simulink model "FYP_Flywheel_Stage1"  (R2024a)
settings: Solver=ode45  StartTime=0.0  StopTime=10  RelTol=1e-3
values from neighbouring files (symbols this model uses):
  J = 0.5    [FYP_Flywheel_Stage1_build.m]    (also in FYP_Flywheel_Stage2_build.m)
  omega0 = 2*pi*n0/60    (= 314.159265359)    [FYP_Flywheel_Stage1_build.m]    (also in FYP_Flywheel_Stage2_build.m; FYP_Flywheel_Stage3_DCServo_build.m; FYP_Flywheel_Stage4_v2_StableClosedLoop_build.m; FYP_Flywheel_Stage5_COMPLETE_v2.m)
settings Model: Creator=cheng  LastModifiedBy=cheng

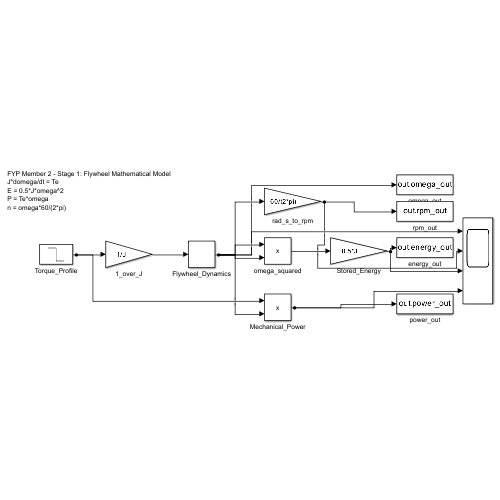
[thumbnail: Simulink's stored preview of the top-level diagram]
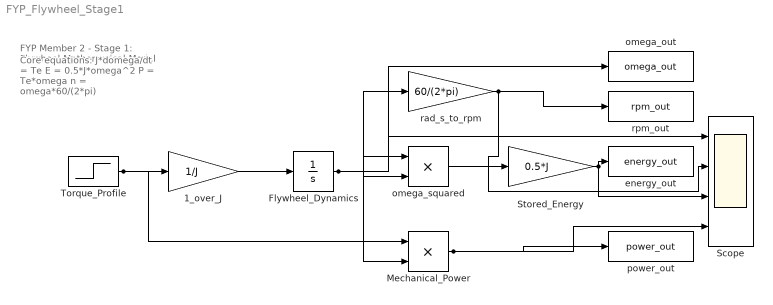
== system FYP_Flywheel_Stage1 ==
  note: FYP Member 2 - Stage 1: Flywheel Mathematical Model
  note: Core equations:
      | J*domega/dt = Te
      | E = 0.5*J*omega^2
      | P = Te*omega
      | n = omega*60/(2*pi)
  1_over_J : Gain  Gain=1/J
  Flywheel_Dynamics : Integrator  InitialCondition=omega0
  Mechanical_Power : Product  Inputs=**
  Scope : Scope  NumInputPorts=4
  Stored_Energy : Gain  Gain=0.5*J
  Torque_Profile : Step  Time=5  Before=5  After=-5  SampleTime=0
  energy_out : ToWorkspace  VariableName=energy_out  SaveFormat=Timeseries  SampleTime=-1
  omega_out : ToWorkspace  VariableName=omega_out  SaveFormat=Timeseries  SampleTime=-1
  omega_squared : Product  Inputs=**
  power_out : ToWorkspace  VariableName=power_out  SaveFormat=Timeseries  SampleTime=-1
  rad_s_to_rpm : Gain  Gain=60/(2*pi)
  rpm_out : ToWorkspace  VariableName=rpm_out  SaveFormat=Timeseries  SampleTime=-1
  wires:
  Torque_Profile/1 -> 1_over_J/1, Mechanical_Power/1
  1_over_J/1 -> Flywheel_Dynamics/1
  Flywheel_Dynamics/1 -> rad_s_to_rpm/1, omega_squared/1, omega_squared/2, Mechanical_Power/2, omega_out/1, Scope/1
  omega_squared/1 -> Stored_Energy/1
  rad_s_to_rpm/1 -> rpm_out/1, Scope/2
  Stored_Energy/1 -> energy_out/1, Scope/3
  Mechanical_Power/1 -> power_out/1, Scope/4
